simulink model "Model_7"  (Simulink 8.6)
settings: Solver=ode4  StartTime=0.0  StopTime=2000  FixedStep=1  RelTol=1e-3
settings Model: Creator=josegarcia  LastModifiedBy=Kazemiro
settings DataIOCC: SignalLoggingSaveFormat=Dataset
settings OptimizationCC: ExpressionDepthLimit=128
settings DebuggingCC: UnderspecifiedInitializationDetection=Simplified  MergeDetectMultiDrivingBlocksExec=error  SolverPrmCheckMsg=none  FcnCallInpInsideContextMsg=EnableAllAsError  StateNameClashWarn=none
settings GRTTargetCC: CombineOutputUpdateFcns=on  GRTInterface=off

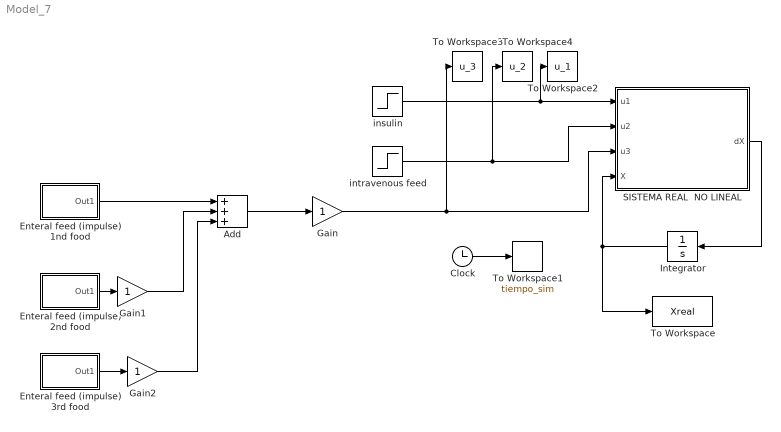
== system Model_7 ==
  Add : Sum  Inputs=+++
  Clock : Clock
  Enteral feed (impulse) 1nd food : Subsystem  mask{t1=420, t2=40, Am=5.55, Am_b=0}
      mask prompts: t1 "Impulse time (min)"; t2 "Impulse duration (min)"; Am "Impulse amplitude (mmol/min)"; Am_b "Basal input (mmol/min)"
  Enteral feed (impulse) 2nd food : Subsystem  mask{t1=780, t2=40, Am=5.55, Am_b=0}
      mask prompts: t1 "Impulse time (min)"; t2 "Impulse duration (min)"; Am "Impulse amplitude (mmol/min)"; Am_b "Basal input (mmol/min)"
  Enteral feed (impulse) 3rd food : Subsystem  mask{t1=1140, t2=40, Am=5.55, Am_b=0}
      mask prompts: t1 "Impulse time (min)"; t2 "Impulse duration (min)"; Am "Impulse amplitude (mmol/min)"; Am_b "Basal input (mmol/min)"
  Gain : Gain
  Gain1 : Gain
  Gain2 : Gain
  Integrator : Integrator  InitialCondition=[5 5 74 108.58 0 0]'
  SISTEMA REAL  NO LINEAL : MATLAB Function  TreatAsAtomicUnit=on
  To Workspace : ToWorkspace  VariableName=Xreal  SampleTime=-1
  To Workspace1 : ToWorkspace  VariableName=tiempo_sim  SampleTime=-1
      settings: Save2DSignal=2-D array (concatenate along first dimension)
  To Workspace2 : ToWorkspace  VariableName=u_1  SampleTime=-1
      settings: Save2DSignal=2-D array (concatenate along first dimension)
  To Workspace3 : ToWorkspace  VariableName=u_3  SampleTime=-1
      settings: Save2DSignal=2-D array (concatenate along first dimension)
  To Workspace4 : ToWorkspace  VariableName=u_2  SampleTime=-1
      settings: Save2DSignal=2-D array (concatenate along first dimension)
  insulin : Step  Before=58.91  After=58.91  SampleTime=0  VectorParams1D=off
  intravenous feed : Step  After=0  SampleTime=0  VectorParams1D=off
  wires:
  SISTEMA REAL  NO LINEAL/1(dX) -> Integrator/1
  insulin/1 -> To Workspace2/1, SISTEMA REAL  NO LINEAL/1(u1)
  Integrator/1 -> To Workspace/1, SISTEMA REAL  NO LINEAL/4(X)
  intravenous feed/1 -> SISTEMA REAL  NO LINEAL/2(u2), To Workspace4/1
  Gain/1 -> To Workspace3/1, SISTEMA REAL  NO LINEAL/3(u3)
  Clock/1 -> To Workspace1/1
  Enteral feed (impulse) 2nd food/1(Out1) -> Gain1/1
  Enteral feed (impulse) 3rd food/1(Out1) -> Gain2/1
  Add/1 -> Gain/1
  Enteral feed (impulse) 1nd food/1(Out1) -> Add/1
  Gain1/1 -> Add/2
  Gain2/1 -> Add/3

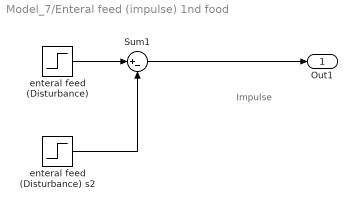
== system Model_7/Enteral feed (impulse) 1nd food ==
  note: Impulse
  Sum1 : Sum  Inputs=|+-
  enteral feed (Disturbance) : Step  Time=t1  Before=Am_b  After=Am  SampleTime=0  VectorParams1D=off
  enteral feed (Disturbance) s2 : Step  Time=t1+t2  After=Am-Am_b  SampleTime=0  VectorParams1D=off
  Out1 : Outport
  wires:
  enteral feed (Disturbance)/1 -> Sum1/1
  enteral feed (Disturbance) s2/1 -> Sum1/2
  Sum1/1 -> Out1/1

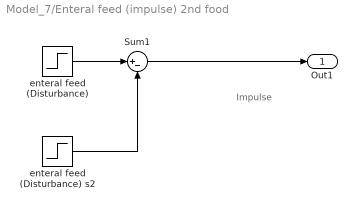
== system Model_7/Enteral feed (impulse) 2nd food ==
  note: Impulse
  Sum1 : Sum  Inputs=|+-
  enteral feed (Disturbance) : Step  Time=t1  Before=Am_b  After=Am  SampleTime=0  VectorParams1D=off
  enteral feed (Disturbance) s2 : Step  Time=t1+t2  After=Am-Am_b  SampleTime=0  VectorParams1D=off
  Out1 : Outport
  wires:
  Sum1/1 -> Out1/1
  enteral feed (Disturbance) s2/1 -> Sum1/2
  enteral feed (Disturbance)/1 -> Sum1/1

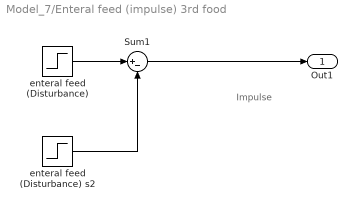
== system Model_7/Enteral feed (impulse) 3rd food ==
  note: Impulse
  Sum1 : Sum  Inputs=|+-
  enteral feed (Disturbance) : Step  Time=t1  Before=Am_b  After=Am  SampleTime=0  VectorParams1D=off
  enteral feed (Disturbance) s2 : Step  Time=t1+t2  After=Am-Am_b  SampleTime=0  VectorParams1D=off
  Out1 : Outport
  wires:
  enteral feed (Disturbance)/1 -> Sum1/1
  enteral feed (Disturbance) s2/1 -> Sum1/2
  Sum1/1 -> Out1/1

== matlab function SISTEMA REAL NO LINEAL ==
  data: u1 input double; dX output double; u2 input double; u3 input double; X input double
function dX = fcn(u1,u2,u3,X)
%#codegen

BG = X(1);
Gi = X(2);
Q = X(3);
I = X(4);
P1 = X(5);
P2 = X(6);

uex = u1;           % [mU/min]
PN = u2;            % [mmol/min]
D = u3;             % [mmol/min]

% Parameters
pG = 0.006;         % Patient endogenous glucose removal [min^-1]
Si = 0.0002;         % From former model since it is identified online [L/mU/min]
aG = 0.0154;        % Saturation of insulin-stimulated glucose [L/mU]
EGPb = 1.16;        % Basal endogenous glucose production [mmol/min]
CNS = 0.3;          % Insulin independent central nervous system glucose uptake [mmol/min]
VG = 13.3;          % Glucose distribution volume [L]
VI = 3.15;          % Insulin distribution volume [L]
aI = 0.0017;        % Saturation of plasma insulin disappearance [L/mU]
nI = 0.003;         % Transcapillary difussion rate [min^-1]
nC = nI;            % [min^-1]
nK = 0.0542;        % Kidney clearance [min^-1]
nL = 0.1578;        % Patient specific liver clearance [min^-1]
xL = 0.67;          % First pass endogenous insulin hepatic uptake []
d1 = 0.0347;        % Transport rate [min^-1]
d2 = 0.0069;        % Transport rate [min^-1]
Pmax = 6.11;        % Saturation value of P2 [mmol/min]
k1 = 45.7;          % Base rate for endogenous insulin production [mU/min]
k2 = 1.5;           % Generic constant for exponential supression []
k3 = 1000;          % Generic constant for exponential supression []
beta1=0.09;
beta2=beta1;

P = min(d2*P2,Pmax) + PN;
uen = k1*exp(-I^(k2/k3));

dBG = -pG*BG - Si*BG*Q/(1 + aG*Q) + (P + EGPb - CNS)/VG;
dGi=beta1*BG-beta2*Gi;
dQ = nI*(I - Q) - nC*Q/(1 + aG*Q);
dI = -nK*I - nL*I/(1 + aI*I) - nI*(I - Q) + uex/VI + (1 - xL)*uen/VI;
dP1 = -d1*P1 + D;
dP2 = -min(d2*P2,Pmax) + d1*P1;

dX = [dBG dGi dQ dI dP1 dP2]';
